simulink model "CoVM_TrqDesCoord"  (R2018a)
settings: configuration reference "cs_ert" (kept outside this file)
settings Model: DataDictionary=CoVM_TrqDesCoord.sldd  Creator=zhoutinglin  LastModifiedBy=zhoutinglin

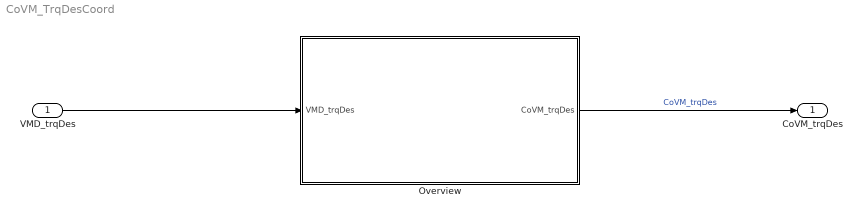
== system CoVM_TrqDesCoord ==
  VMD_trqDes : Inport  Description="propulsion  torque after driving assistance coordination"  OutMin=-3000  OutMax=3000  OutDataTypeStr=Torq  Unit=Nm  PortDimensions=[1 1]
  Overview : Subsystem
  CoVM_trqDes : Outport
  wires:
  VMD_trqDes/1 -> Overview/1(VMD_trqDes)
  Overview/1(CoVM_trqDes) -> CoVM_trqDes/1  "CoVM_trqDes"

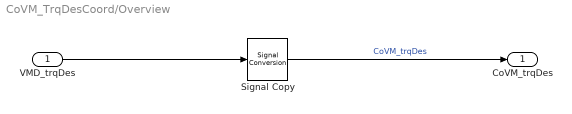
== system CoVM_TrqDesCoord/Overview ==
  VMD_trqDes : Inport  Tag=Nm
  Signal Copy : SignalConversion  OverrideOpt=off
  CoVM_trqDes : Outport  Tag=Nm
  wires:
  Signal Copy/1 -> CoVM_trqDes/1  "CoVM_trqDes"
  VMD_trqDes/1 -> Signal Copy/1
